simulink model "MATMPC_SIMULINK_SPACEROBOT"  (R2019b)
settings: Solver=ode1  StartTime=0.0  StopTime=10  FixedStep=settings.Ts  RelTol=1e-3
undefined symbols (not defined in the file): indata, opt, settings, x0
libraries: dspindex x3
(part 2 of 2)

== matlab function MATMPC_SIMULINK_SPACEROBOT/NMPC Controller/Parameters_Checker ==
  data: para output size=settings.size_od; settings parameter; input input; z_0 output
function [para, z_0]  = Parameters_Checker(settings, input)
% PARA_GENERATOR Prepares para matrix for NMPC solver. 
%
% Para is a matrix containing all the params values over all shooting
% points. Each column j is a vector containing params values for the j-th
% shooting point. Therefore the para matrix must have the number of rows
% equal to the number of params and number of columns equal to N+1, where N
% is the number of shooting points.
%
%   para PARA_GENERATOR(input, settings)
%     
%     Inputs:
%     ---------------------------------------------------------------------
%       - input: struct containing all params. Each field is a different
%                param
%
%       - settings: struct containing data related to the settings used in
%                   the simulation
%           -> Ts: sampling time [s] (i.e. time at which the controller
%                  works)
%           -> Ts_st: shooting interval [s], i.e. temporal distance between 
%                     one shooting point and the next one
%           -> s: number of integration steps per interval
%           -> nx: no. of states
%           -> nu: no. of controls
%           -> ny: no. of outputs (references)    
%           -> nyN: no. of outputs at terminal stage 
%           -> np: no. of parameters (on-line data)
%           -> nc: no. of constraints
%           -> ncN: no. of constraints at terminal stage
%           -> nbu: no. of control bounds
%           -> nbx: no. of state bounds
%           -> nbu_idx: index of control bounds
%           -> nbx_idx: index of state bounds
%           -> N: no. of shooting points
%           -> N2: no. of partial condensing blocks 
%           -> r: no. of input move blocks
%
%     Outputs:
%     ---------------------------------------------------------------------
%       - para: matrix containing all the params values over all shooting
%               points. Each column j is a vector containing params values 
%               for the j-th shooting point. Its dimension is
%               [no_of_params, N+1], where N is the number of shooting
%               points

    %% Extracting variables from settings struct
    
    % Number of shooting points
    N = settings.N;
    np = settings.np;
    nz = settings.nz;
    %% Arraging params in para vector
    % para must be a matrix, where each column j is the vector of params of
    % the j-th shooting point
    
    if np > 0
        input_rows = size(input, 1);
        input_columns = size(input, 2);
        if input_rows == np && input_columns == N+1
            para = input;
        else
            error('NMPC para vector has invalid size!');
        end
    else
        para = zeros(1, N+1); % see settings.size_od
    end
    z_0 = settings.z0;
     % faire un bloc espace algebrique 
    % Sice at the beginning of the NMPC solver this param is constant over
    % all shooting points, replicate it over n+1 column
%     para = repmat(params, 1, N+1); % dimension = [n_of_params, N+1], where N is the number of shooting points
end

== matlab function MATMPC_SIMULINK_SPACEROBOT/NMPC Controller/Weights_SubSystem/Weights_Gen ==
  settings: sampleTime=sim_time_step
  data: W output size=settings.size_W; settings parameter; indata parameter; states input size=settings.nx; WN output size=settings.size_WN
function [W, WN]  = Weights_Gen(settings, indata, states)
%% Importing variables 
% ... from parameter `settings`
nyN = settings.nyN;
N = settings.N;

% ... from parameter `data`
q = indata.weights.q;

% ... from input `states`

%% Do something here

%% Format correctly weights for the cost function
W = repmat(q', 1, N);
WN = W(1:nyN, 1);
